simulink model "EE307_Simulink_Model"  (R2022a)
settings: Solver=ode45  StartTime=0.0  StopTime=2.0  MaxStep=1e-6  MinStep=1e-7  RelTol=1e-3
libraries: simulink x1, cstblocks x1
settings Model: Creator=Lenovo  LastModifiedBy=Lenovo

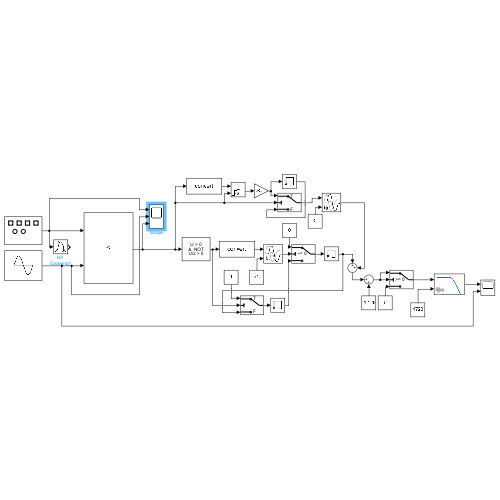
[thumbnail: Simulink's stored preview of the top-level diagram]
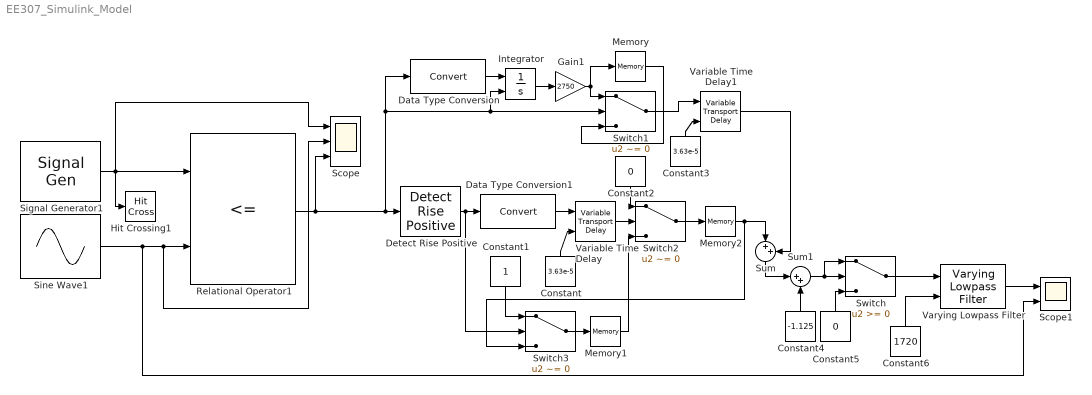
== system EE307_Simulink_Model ==
  Constant : Constant  Value=3.63e-5
  Constant1 : Constant
  Constant2 : Constant  Value=0
  Constant3 : Constant  Value=3.63e-5
  Constant4 : Constant  Value=-1.125
  Constant5 : Constant  Value=0
  Constant6 : Constant  Value=1720
  Data Type Conversion : DataTypeConversion  SaturateOnIntegerOverflow=off  RndMeth=Floor
  Data Type Conversion1 : DataTypeConversion  SaturateOnIntegerOverflow=off  RndMeth=Floor
  Detect Rise Positive : simulink/Logic and Bit Operations/Detect Rise Positive  vinit=0  OutDataTypeStr=boolean
  Gain1 : Gain  Gain=2750
  Hit Crossing1 : HitCross
  Integrator : Integrator  ExternalReset=rising
  Memory : Memory
  Memory1 : Memory
  Memory2 : Memory
  Relational Operator1 : RelationalOperator  Operator=<=  OutDataTypeStr=boolean  RndMeth=Simplest  InputSameDT=off
  Scope : Scope  NumInputPorts=3
  Scope1 : Scope  NumInputPorts=2
  Signal Generator1 : SignalGenerator  WaveForm=sawtooth  Frequency=2750  VectorParams1D=off
  Sine Wave1 : Sin  Amplitude=0.75  Frequency=20*pi  SampleTime=0
  Sum : Sum  Inputs=|++
  Sum1 : Sum  Inputs=|++
  Switch : Switch  SaturateOnIntegerOverflow=off  InputSameDT=off
  Switch1 : Switch  Criteria=u2 ~= 0  SaturateOnIntegerOverflow=off  InputSameDT=off
  Switch2 : Switch  Criteria=u2 ~= 0  Threshold=40000  SaturateOnIntegerOverflow=off  InputSameDT=off
  Switch3 : Switch  Criteria=u2 ~= 0  Threshold=40000  SaturateOnIntegerOverflow=off  InputSameDT=off
  Variable Time Delay : VariableTransportDelay  MaximumDelay=10
  Variable Time Delay1 : VariableTransportDelay  MaximumDelay=10
  Varying Lowpass Filter : cstblocks/Linear Parameter Varying/Varying Lowpass Filter  N=5
  wires:
  Sine Wave1/1 -> Scope1/2, Scope/2, Relational Operator1/2
  Signal Generator1/1 -> Scope/1, Hit Crossing1/1, Relational Operator1/1
  Data Type Conversion/1 -> Integrator/1
  Integrator/1 -> Gain1/1
  Memory/1 -> Switch1/3
  Gain1/1 -> Memory/1, Switch1/1
  Relational Operator1/1 -> Detect Rise Positive/1, Data Type Conversion/1, Integrator/2, Switch1/2, Scope/3
  Data Type Conversion1/1 -> Variable Time Delay/1
  Detect Rise Positive/1 -> Switch3/2, Data Type Conversion1/1
  Constant/1 -> Variable Time Delay/2
  Constant2/1 -> Switch2/1
  Constant1/1 -> Switch3/1
  Switch3/1 -> Memory1/1
  Memory1/1 -> Switch2/3
  Variable Time Delay/1 -> Switch2/2
  Switch2/1 -> Memory2/1
  Memory2/1 -> Switch3/3, Sum/1
  Sum/1 -> Sum1/1
  Switch1/1 -> Variable Time Delay1/1
  Constant3/1 -> Variable Time Delay1/2
  Variable Time Delay1/1 -> Sum/2
  Constant4/1 -> Sum1/2
  Sum1/1 -> Switch/1, Switch/2
  Constant5/1 -> Switch/3
  Switch/1 -> Varying Lowpass Filter/1
  Constant6/1 -> Varying Lowpass Filter/2
  Varying Lowpass Filter/1 -> Scope1/1
